simulink model "AUV_Model"  (R2019b)
settings: Solver=VariableStepAuto  StartTime=0.0  StopTime=300  FixedStep=0.5  RelTol=1e-3
InitFcn:
  | mdlWks = get_param(gcs,'ModelWorkspace');
  | a = getVariable(mdlWks,'a');
  | b = getVariable(mdlWks,'b');
  | c = getVariable(mdlWks,'c');
StopFcn:
  | figure(2)
  | plot3(Position_Data(1,1),Position_Data(1,2),Position_Data(1,3),'r*')
  | hold on
  | plot3(Position_Data(:,1),Position_Data(:,2),Position_Data(:,3));
  | plot3(Position_Data(end,1),Position_Data(end,2),Position_Data(end,3),'g*');
  | grid on
  | legend('Start Point','Trajectory','End Point')
model workspace (MAT data in the model file):
  a = 1
  b = 0
  c = 1
undefined symbols (not defined in the file): sigbuilder_block
libraries: simulink x6, sharedtransform x6, vrlib x6, dspfdesign x6, shared6dof x1, aerolibasang x1, aerolibnav x1
(part 1 of 3)
settings Model: EnablePacing=on  ParameterArgumentNames=a  OrderedModelArguments=off  Creator=yveerall  LastModifiedBy=cdsouza
settings DataIOCC: ReturnWorkspaceOutputs=off
settings DebuggingCC: ArithmeticOperatorsInVariantConditions=warning
settings SFSimCC: CustomCodeUndefinedFunction=UseInterfaceOnly

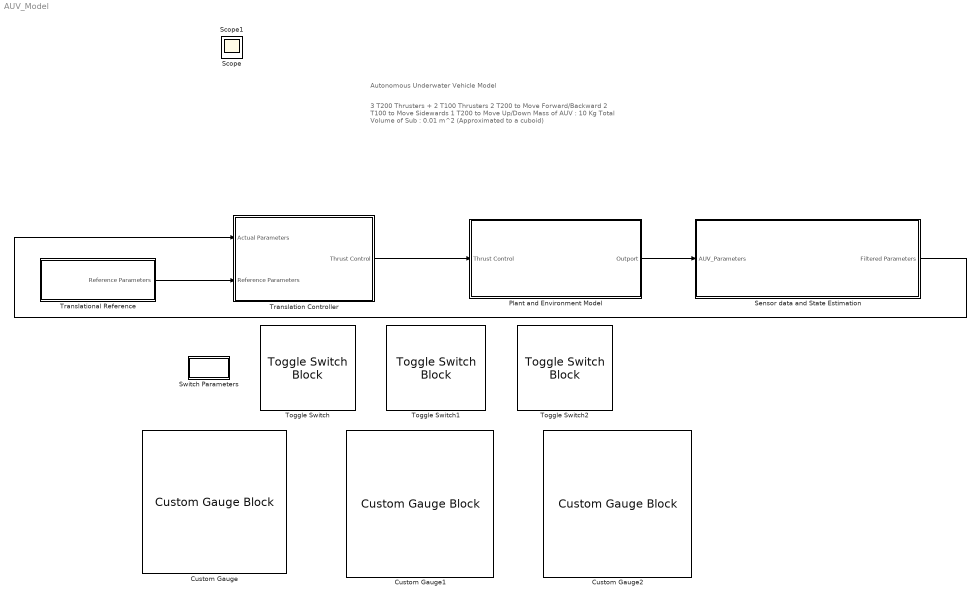
== system AUV_Model ==
  note: Autonomous Underwater Vehicle Model
  note: 3 T200 Thrusters + 2 T100 Thrusters
      |
      | 2 T200 to Move Forward/Backward
      | 2 T100 to Move Sidewards
      | 1 T200 to Move Up/Down
      |
      | Mass of AUV : 10 Kg
      | Total Volume of Sub : 0.01 m^2 (Approximated to a cuboid)
  " Translation Controller" : Subsystem  Variant=on
  Custom Gauge : CustomGaugeBlock  NeedleImage=data:image/svg+xml;base64,PD94bWwgdmVyc2lvbj0iMS4wIiBlbmNvZGluZz0idXRmLTgiPz4KPCEtLSBHZW5lcmF0b3I6IEFkb2JlIElsbHVzdHJhdG9yIDE5LjIuMSwgU1ZHIEV4cG9ydCBQbHVnLUluIC4gU1ZHIFZlcnNpb246IDYuMDAgQnVpbGQgMCkgIC0tPgo8c3ZnIHZlcnNpb249IjEuMSIgeG1sbnM9Imh0dHA6Ly93d3cudzMub3JnLzIwMDAvc3ZnIiB4bWxuczp4bGluaz0iaHR0cDovL3d3dy53My5vcmcvMTk5OS94bGluayIgeD0iMHB4IiB5PSIwcHgiCgkgdmlld0JveD0iMCAwIDIwMCA1MCIgc3R5bGU9ImVuYWJsZS1iYWNrZ3JvdW5kOm5ldyAw ...(+9940 chars)  NeedleXPos=0.38265380737030785  NeedleYPos=0.4815540899511936  NeedleHeight=0.11367340007583818  NeedleWidth=0.1872685327639379  NeedleInitialRotation=-59.94322499147643  BackgroundImage=data:image/svg+xml;base64,PD94bWwgdmVyc2lvbj0iMS4wIiBlbmNvZGluZz0iVVRGLTgiIHN0YW5kYWxvbmU9Im5vIj8+CjwhLS0gR2VuZXJhdG9yOiBBZG9iZSBJbGx1c3RyYXRvciAxOS4yLjEsIFNWRyBFeHBvcnQgUGx1Zy1JbiAuIFNWRyBWZXJzaW9uOiA2LjAwIEJ1aWxkIDApICAtLT4KCjxzdmcKICAgeG1sbnM6ZGM9Imh0dHA6Ly9wdXJsLm9yZy9kYy9lbGVtZW50cy8xLjEvIgogICB4bWxuczpjYz0iaHR0cDovL2NyZWF0aXZlY29tbW9ucy5vcmcvbnMjIgogICB4bWxuczpyZGY9Imh0dHA6Ly93d3cudzMub3JnLzE5OTkvMDIvMjItcmRmLXN5bnRh ...(+9660 chars)  GaugeMin=-1  GaugeMax=+1  GaugeArcDefined=true  GaugeArcRadius=0.13310683978787397  GaugeArcStrokeWidth=0.03892557816851485  GaugeArcRotation=240.5385250290321  GaugeArcRatio=0.8333333333333  GaugeArcTransparency=0  ValueArcColor=#1759b0  GaugeTickColor=#faf5c8  ScaleColorsJSON=[]  fixedAspectRatio=on  IsLinearGauge=false  GaugeTrackLeft=0.35  GaugeTrackTop=0.35  GaugeTrackHeight=0.1  GaugeTrackWidth=0.3  GaugeTrackRotation=0  ScaleMin=-1
  Custom Gauge1 : CustomGaugeBlock  NeedleImage=data:image/svg+xml;base64,PD94bWwgdmVyc2lvbj0iMS4wIiBlbmNvZGluZz0idXRmLTgiPz4KPCEtLSBHZW5lcmF0b3I6IEFkb2JlIElsbHVzdHJhdG9yIDE5LjIuMSwgU1ZHIEV4cG9ydCBQbHVnLUluIC4gU1ZHIFZlcnNpb246IDYuMDAgQnVpbGQgMCkgIC0tPgo8c3ZnIHZlcnNpb249IjEuMSIgeG1sbnM9Imh0dHA6Ly93d3cudzMub3JnLzIwMDAvc3ZnIiB4bWxuczp4bGluaz0iaHR0cDovL3d3dy53My5vcmcvMTk5OS94bGluayIgeD0iMHB4IiB5PSIwcHgiCgkgdmlld0JveD0iMCAwIDIwMCA1MCIgc3R5bGU9ImVuYWJsZS1iYWNrZ3JvdW5kOm5ldyAw ...(+9940 chars)  NeedleXPos=0.3840747354172573  NeedleYPos=0.48177744880376894  NeedleHeight=0.11229694534185655  NeedleWidth=0.18500092522975004  NeedleInitialRotation=-59.94322499147643  BackgroundImage=data:image/svg+xml;base64,PD94bWwgdmVyc2lvbj0iMS4wIiBlbmNvZGluZz0iVVRGLTgiIHN0YW5kYWxvbmU9Im5vIj8+CjwhLS0gR2VuZXJhdG9yOiBBZG9iZSBJbGx1c3RyYXRvciAxOS4yLjEsIFNWRyBFeHBvcnQgUGx1Zy1JbiAuIFNWRyBWZXJzaW9uOiA2LjAwIEJ1aWxkIDApICAtLT4KCjxzdmcKICAgeG1sbnM6ZGM9Imh0dHA6Ly9wdXJsLm9yZy9kYy9lbGVtZW50cy8xLjEvIgogICB4bWxuczpjYz0iaHR0cDovL2NyZWF0aXZlY29tbW9ucy5vcmcvbnMjIgogICB4bWxuczpyZGY9Imh0dHA6Ly93d3cudzMub3JnLzE5OTkvMDIvMjItcmRmLXN5bnRh ...(+9660 chars)  GaugeMin=-1  GaugeMax=+1  GaugeArcDefined=true  GaugeArcRadius=0.13149506834768554  GaugeArcStrokeWidth=0.03845423398150822  GaugeArcRotation=240.5385250290321  GaugeArcRatio=0.8333333333333  GaugeArcTransparency=0  ValueArcColor=#1759b0  GaugeTickColor=#faf5c8  ScaleColorsJSON=[]  fixedAspectRatio=on  IsLinearGauge=false  GaugeTrackLeft=0.35  GaugeTrackTop=0.35  GaugeTrackHeight=0.1  GaugeTrackWidth=0.3  GaugeTrackRotation=0  ScaleMin=-1
  Custom Gauge2 : CustomGaugeBlock  NeedleImage=data:image/svg+xml;base64,PD94bWwgdmVyc2lvbj0iMS4wIiBlbmNvZGluZz0idXRmLTgiPz4KPCEtLSBHZW5lcmF0b3I6IEFkb2JlIElsbHVzdHJhdG9yIDE5LjIuMSwgU1ZHIEV4cG9ydCBQbHVnLUluIC4gU1ZHIFZlcnNpb246IDYuMDAgQnVpbGQgMCkgIC0tPgo8c3ZnIHZlcnNpb249IjEuMSIgeG1sbnM9Imh0dHA6Ly93d3cudzMub3JnLzIwMDAvc3ZnIiB4bWxuczp4bGluaz0iaHR0cDovL3d3dy53My5vcmcvMTk5OS94bGluayIgeD0iMHB4IiB5PSIwcHgiCgkgdmlld0JveD0iMCAwIDIwMCA1MCIgc3R5bGU9ImVuYWJsZS1iYWNrZ3JvdW5kOm5ldyAw ...(+9940 chars)  NeedleXPos=0.3870364203843521  NeedleYPos=0.48224300267707054  NeedleHeight=0.10942795749812154  NeedleWidth=0.18027447960873946  NeedleInitialRotation=-59.94322499147643  BackgroundImage=data:image/svg+xml;base64,PD94bWwgdmVyc2lvbj0iMS4wIiBlbmNvZGluZz0iVVRGLTgiIHN0YW5kYWxvbmU9Im5vIj8+CjwhLS0gR2VuZXJhdG9yOiBBZG9iZSBJbGx1c3RyYXRvciAxOS4yLjEsIFNWRyBFeHBvcnQgUGx1Zy1JbiAuIFNWRyBWZXJzaW9uOiA2LjAwIEJ1aWxkIDApICAtLT4KCjxzdmcKICAgeG1sbnM6ZGM9Imh0dHA6Ly9wdXJsLm9yZy9kYy9lbGVtZW50cy8xLjEvIgogICB4bWxuczpjYz0iaHR0cDovL2NyZWF0aXZlY29tbW9ucy5vcmcvbnMjIgogICB4bWxuczpyZGY9Imh0dHA6Ly93d3cudzMub3JnLzE5OTkvMDIvMjItcmRmLXN5bnRh ...(+9660 chars)  GaugeMin=-1  GaugeMax=+1  GaugeArcDefined=true  GaugeArcRadius=0.12813560250066575  GaugeArcStrokeWidth=0.03747179648512543  GaugeArcRotation=240.5385250290321  GaugeArcRatio=0.8333333333333  GaugeArcTransparency=0  ValueArcColor=#1759b0  GaugeTickColor=#faf5c8  ScaleColorsJSON=[]  fixedAspectRatio=on  IsLinearGauge=false  GaugeTrackLeft=0.35  GaugeTrackTop=0.35  GaugeTrackHeight=0.1  GaugeTrackWidth=0.3  GaugeTrackRotation=0  ScaleMin=-1
  Plant and Environment Model : Subsystem
  Sensor data and State Estimation : Subsystem  Variant=on
  Switch Parameters : Subsystem
      mask Display: text(0.5, 0.5, 'Switch Parameters', 'horizontalAlignment', 'center')
  Toggle Switch : ToggleSwitchBlock
      settings: Values={{'Velocity Control', 'Position Control'}, [1 0]}
  Toggle Switch1 : ToggleSwitchBlock
      settings: Values={{'Low Fidelity Simulation', 'High Fidelity Simulation'}, [0 1]}
  Toggle Switch2 : ToggleSwitchBlock
      settings: Values={{'System with Noise', 'System without Noise'}, [0 1]}
  Translational Reference : Subsystem
  Scope : Scope
  Scope1 : Scope
  wires:
  Translational Reference/1(Reference Parameters) -> " Translation Controller"/2(Reference Parameters)
  " Translation Controller"/1(Thrust Control) -> Plant and Environment Model/1(Thrust Control)
  Plant and Environment Model/1(Outport) -> Sensor data and State Estimation/1(AUV_Parameters)
  Sensor data and State Estimation/1(Filtered Parameters) -> " Translation Controller"/1(Actual Parameters)
